simulink model "PipeModel"  (R2020a)
settings: Solver=ode3  StartTime=0.0  StopTime=100  FixedStep=delta_t  RelTol=1e-3
settings Model: Creator=saif  LastModifiedBy=Afraz
settings DataIOCC: LimitDataPoints=on  SaveFormat=Array  ReturnWorkspaceOutputs=off
settings OptimizationCC: BlockReduction=off  BooleanDataType=off  LifeSpan=inf
settings DebuggingCC: SaveWithParameterizedLinksMsg=none  UnderspecifiedInitializationDetection=Classic  MergeDetectMultiDrivingBlocksExec=none  SignalResolutionControl=TryResolveAllWithWarning  SFUnexpectedBacktrackingDiag=warning  SFNoUnconditionalDefaultTransitionDiag=warning  ArithmeticOperatorsInVariantConditions=warning
settings HardwareCC: ProdBitPerPointer=32  ProdBitPerSizeT=32  ProdBitPerPtrDiffT=32  ProdLargestAtomicFloat=None  ProdIntDivRoundTo=Undefined  ProdEndianess=Unspecified  ProdWordSize=32  ProdHWDeviceType=32-bit Generic  TargetUnknown=on
settings ModelReferenceCC: PropagateSignalLabelsOutOfModel=off
settings SFSimCC: SimUseLocalCustomCode=off  CustomCodeUndefinedFunction=UseInterfaceOnly
settings RTWCC: RTWUseLocalCustomCode=off
settings CodeAppCC: StateflowObjectComments=on
settings GRTTargetCC: TargetLangStandard=C89/C90 (ANSI)
settings ConfigComp: CovMetricSettings=dw  CovHtmlReporting=on  CovSaveCumulativeToWorkspaceVar=on  CovSaveSingleToWorkspaceVar=on  CovExternalEMLEnable=off  CovSFcnEnable=off

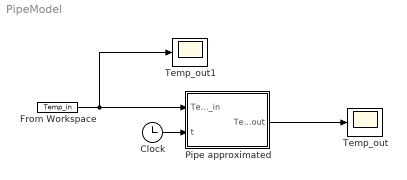
== system PipeModel ==
  Clock : Clock
  From Workspace : FromWorkspace  VariableName=Temp_in  SampleTime=-1
  Pipe approximated : Subsystem
  Temp_out : Scope
  Temp_out1 : Scope
  wires:
  From Workspace/1 -> Temp_out1/1, Pipe approximated/1(Temp_in)
  Clock/1 -> Pipe approximated/2(t)
  Pipe approximated/1(Temp_out) -> Temp_out/1

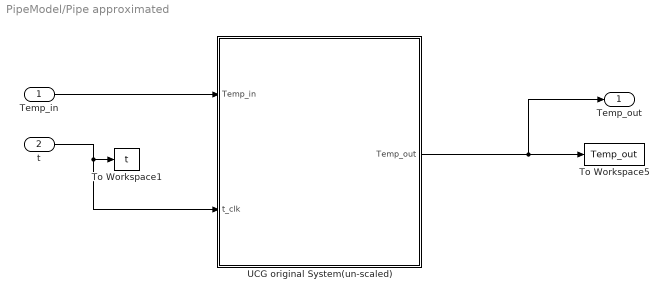
== system PipeModel/Pipe approximated ==
  Temp_in : Inport
  t : Inport  Port=2
  To Workspace1 : ToWorkspace  VariableName=t  SampleTime=-1
  To Workspace5 : ToWorkspace  VariableName=Temp_out  SampleTime=-1
  UCG original System(un-scaled) : MATLAB Function  TreatAsAtomicUnit=on
  Temp_out : Outport
  wires:
  UCG original System(un-scaled)/1(Temp_out) -> Temp_out/1, To Workspace5/1
  t/1 -> To Workspace1/1, UCG original System(un-scaled)/2(t_clk)
  Temp_in/1 -> UCG original System(un-scaled)/1(Temp_in)

== matlab function PipeModel/Pipe approximated/UCG original System(un-scaled) ==
  data: Temp_in input; t_clk input; Temp_out output; param parameter
function Temp_out  = fcn(Temp_in,t_clk, param)
%#codegen
% param=[rho Cp_w L D_ins_out Tb K D_steel_out D_steel_in flowrate A v delay R_tot RC length_t Temp_ramp];
% Temp_out=273*ones(1,param(15));
% Temp_out=273.15*ones(1,1);
% for i=(param(12)+1):1:length(param(15))
Temp_out=273.15*ones(1,1)
    if t_clk<param(16)+param(12)  
        Temp_out=273.15;
    else
Temp_out= param(5)+(Temp_in-param(5))*exp(-param(12)/param(14));
 end

% Temp_out=Temp_out;

% dx = [dx1;dx2];
